simulink library "mag_vec_LS_lib"  (R2016b)
settings: Solver=VariableStepAuto  StartTime=0.0  StopTime=10.0  RelTol=1e-3
undefined symbols (not defined in the file or in its folder): fsw_params
libraries: dspmathops x1
settings Model: Creator=taylorreynolds  LastModifiedBy=Taylor

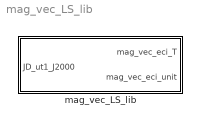
== system mag_vec_LS_lib ==
  mag_vec_LS_lib : Subsystem

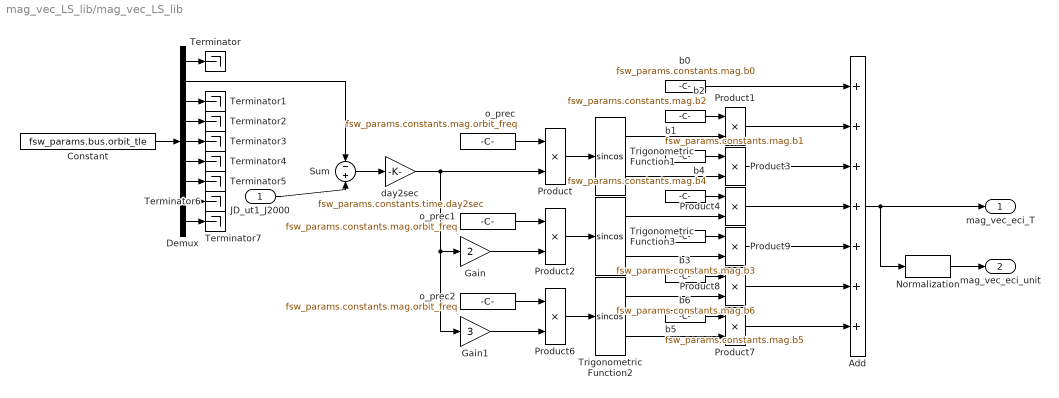
== system mag_vec_LS_lib/mag_vec_LS_lib ==
  JD_ut1_J2000 : Inport
  Add : Sum  Inputs=+++++++
  Constant : Constant  Value=fsw_params.bus.orbit_tle
  Demux : Demux  Outputs=9
  Gain : Gain  Gain=2
  Gain1 : Gain  Gain=3
  Normalization : dspmathops/Normalization  NormType=2-norm  Bias=1e-10  NormOver=Each column  Dimension=1  outputDataTypeStr=Inherit: Same as product output  outputLastDataTypeStr=Inherit: Same as product output  outputMin=[]  outputMax=[]  accumDataTypeStr=Inherit: Same as product output  accumLastDataTypeStr=Inherit: Same as product output  roundingMode=Floor  overflowMode=off
  Product{,1..4,6..9} (9 alike) : Product
  Sum : Sum  Inputs=-+
  Terminator{,1..7} (8 alike) : Terminator
  Trigonometric Function1 : Trigonometry  Operator=sincos
  Trigonometric Function2 : Trigonometry  Operator=sincos
  Trigonometric Function3 : Trigonometry  Operator=sincos
  b0 : Constant  Value=fsw_params.constants.mag.b0
  b1 : Constant  Value=fsw_params.constants.mag.b1
  b2 : Constant  Value=fsw_params.constants.mag.b2
  b3 : Constant  Value=fsw_params.constants.mag.b3
  b4 : Constant  Value=fsw_params.constants.mag.b4
  b5 : Constant  Value=fsw_params.constants.mag.b5
  b6 : Constant  Value=fsw_params.constants.mag.b6
  day2sec : Gain  Gain=fsw_params.constants.time.day2sec
  o_prec : Constant  Value=fsw_params.constants.mag.orbit_freq
  o_prec1 : Constant  Value=fsw_params.constants.mag.orbit_freq
  o_prec2 : Constant  Value=fsw_params.constants.mag.orbit_freq
  mag_vec_eci_T : Outport
  mag_vec_eci_unit : Outport  Port=2
  wires:
  Add/1 -> Normalization/1, mag_vec_eci_T/1
  b0/1 -> Add/1
  o_prec/1 -> Product/1
  Product/1 -> Trigonometric Function1/1
  Product1/1 -> Add/2
  b1/1 -> Product3/1
  b2/1 -> Product1/1
  Product3/1 -> Add/3
  Gain/1 -> Product2/2
  o_prec1/1 -> Product2/1
  Product2/1 -> Trigonometric Function3/1
  Trigonometric Function3/2 -> Product9/2
  b3/1 -> Product9/1
  b4/1 -> Product4/1
  Gain1/1 -> Product6/2
  o_prec2/1 -> Product6/1
  Product6/1 -> Trigonometric Function2/1
  Trigonometric Function2/2 -> Product7/2
  Trigonometric Function2/1 -> Product8/2
  b5/1 -> Product7/1
  b6/1 -> Product8/1
  Trigonometric Function3/1 -> Product4/2
  Trigonometric Function1/2 -> Product3/2
  Trigonometric Function1/1 -> Product1/2
  Product7/1 -> Add/7
  Product8/1 -> Add/6
  Product9/1 -> Add/5
  Product4/1 -> Add/4
  Normalization/1 -> mag_vec_eci_unit/1
  Constant/1 -> Demux/1
  Demux/2 -> Sum/1
  JD_ut1_J2000/1 -> Sum/2
  Sum/1 -> day2sec/1
  day2sec/1 -> Gain1/1, Gain/1, Product/2
  Demux/1 -> Terminator/1
  Demux/3 -> Terminator1/1
  Demux/4 -> Terminator2/1
  Demux/5 -> Terminator3/1
  Demux/6 -> Terminator4/1
  Demux/7 -> Terminator5/1
  Demux/9 -> Terminator7/1
  Demux/8 -> Terminator6/1
